simulink model "SubSnap"  (R2020a)
settings: Solver=FixedStepAuto  StartTime=0.0  StopTime=10.0  FixedStep=0.1  MaxStep=0.1  RelTol=1e-3
settings Model: DataDictionary=TestConfig.sldd  Creator=raarenst  LastModifiedBy=toma
settings OptimizationCC: DefaultParameterBehavior=Inlined  EnhancedBackFolding=on  PassReuseOutputArgsAs=Individual arguments  ZeroExternalMemoryAtStartup=off  ZeroInternalMemoryAtStartup=off  OptimizeBlockOrder=speed  DifferentSizesBufferReuse=on  OptimizationCustomize=off  EfficientTunableParamExpr=on
settings DebuggingCC: UnderspecifiedInitializationDetection=Classic  MergeDetectMultiDrivingBlocksExec=none  ParameterTunabilityLossMsg=error  ModelReferenceSymbolNameMessage=none
settings ModelReferenceCC: PropagateSignalLabelsOutOfModel=off
settings SFSimCC: MATLABDynamicMemAlloc=off
settings RTWCC: Description=CIGRE export target  SystemTargetFile=cigre.tlc  TemplateMakefile=cigre_tmf  Toolchain=CIGRE DLL - Microsoft Visual C++ 2019 (64bit) | nmake makefile (64-bit Windows)
settings CodeAppCC: ForceParamTrailComments=on  IgnoreCustomStorageClasses=off  OperatorAnnotations=on  SimulinkDataObjDesc=on  SFDataObjDesc=on  InsertBlockDesc=on
settings STFCustomTargetCC: TargetLangStandard=C99 (ISO)  MultiwordLength=256  GenerateSampleERTMain=on  CompOptLevelCompliant=on  CombineOutputUpdateFcns=on  ERTCustomFileBanners=on  MultiInstanceERTCode=on  CodeInterfacePackaging=Reusable function  SupportContinuousTime=off  SupportNonInlinedSFcns=off  RemoveResetFunc=on  MATLABClassNameForMDSCustomization=Simulink.SoftwareTarget.ERTCustomization  UseToolchainInfoCompliant=on  SystemTargetFile=cigre.tlc
settings ERTTargetCC: TargetLangStandard=C99 (ISO)  GenerateSampleERTMain=on  ParMdlRefBuildCompliant=off  ConcurrentExecutionCompliant=off  MultiInstanceERTCode=on  CodeInterfacePackaging=Reusable function  ModelStepFunctionPrototypeControlCompliant=off  CPPClassGenCompliant=off  InlinedParameterPlacement=NonHierarchical  RootIOFormat=Structure reference  ERTCustomFileTemplate=example_file_process.tlc

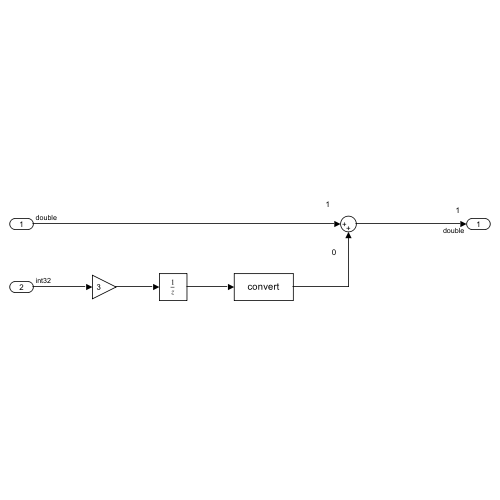
[thumbnail: Simulink's stored preview of the top-level diagram]
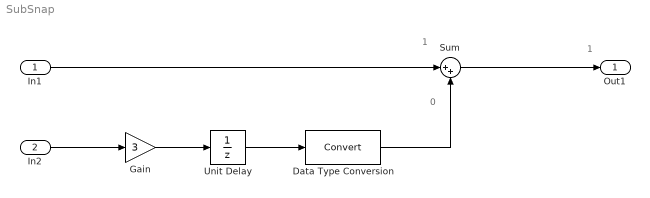
== system SubSnap ==
  note: 0
  note: 1
  note: 1
  In1 : Inport  OutDataTypeStr=double  SampleTime=0.1
  In2 : Inport  Port=2  OutDataTypeStr=int32  SampleTime=0.1
  Data Type Conversion : DataTypeConversion
  Gain : Gain  Gain=3  OutDataTypeStr=int32
  Sum : Sum  Inputs=|++
  Unit Delay : UnitDelay  SampleTime=-1  HasFrameUpgradeWarning=on
  Out1 : Outport  OutDataTypeStr=double
  wires:
  In2/1 -> Gain/1
  Gain/1 -> Unit Delay/1
  Unit Delay/1 -> Data Type Conversion/1
  In1/1 -> Sum/1
  Data Type Conversion/1 -> Sum/2
  Sum/1 -> Out1/1
